simulink model "Ch12_PID_Simulink_Model"  (R2013b)
settings: Solver=ode45  StartTime=0.0  StopTime=100  MaxStep=0.1  RelTol=1e-3
libraries: simulink x1
settings Model: Creator=jeff  LastModifiedBy=jeff
settings DataIOCC: SignalLoggingSaveFormat=ModelDataLogs
settings OptimizationCC: ExpressionDepthLimit=2147483647
settings DebuggingCC: FcnCallInpInsideContextMsg=EnableAllAsWarning  StateNameClashWarn=warning

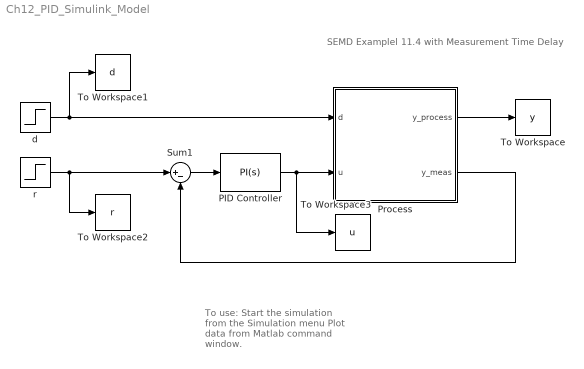
== system Ch12_PID_Simulink_Model ==
  note: SEMD Examplel 11.4 with Measurement Time Delay
  note: To use:
      |     Start the simulation from the Simulation menu
      |     Plot data from Matlab command window.
  PID Controller : simulink/Continuous/PID Controller  Controller=PI  TimeDomain=Continuous-time  SampleTime=1  IntegratorMethod=Forward Euler  FilterMethod=Forward Euler  Form=Ideal  P=1.12313558262161  I=0.142143488109628  D=0  N=100  InitialConditionSource=internal  InitialConditionForIntegrator=0  InitialConditionForFilter=0  ExternalReset=none  LimitOutput=off  UpperSaturationLimit=inf  LowerSaturationLimit=-inf  LinearizeAsGain=off  AntiWindupMode=none  Kb=1  TrackingMode=off  Kt=1  PParamMin=[]  PParamMax=[]  IParamMin=[]  IParamMax=[]  DParamMin=[]  DParamMax=[]  NParamMin=[]  NParamMax=[]  KbParamMin=[]  KbParamMax=[]  KtParamMin=[]  KtParamMax=[]  POutMin=[]  POutMax=[]  IOutMin=[]  IOutMax=[]  DOutMin=[]  DOutMax=[]  NOutMin=[]  NOutMax=[]  KbOutMin=[]  KbOutMax=[]  KtOutMin=[]  KtOutMax=[]  IntegratorOutMin=[]  IntegratorOutMax=[]  FilterOutMin=[]  FilterOutMax=[]  SumOutMin=[]  SumOutMax=[]  SumI1OutMin=[]  SumI1OutMax=[]  SumI2OutMin=[]  SumI2OutMax=[]  SumI3OutMin=[]  SumI3OutMax=[]  SumDOutMin=[]  SumDOutMax=[]  SaturationOutMin=[]  SaturationOutMax=[]  IntegratorContinuousStateAttributes=''  IntegratorStateMustResolveToSignalObject=off  IntegratorRTWStateStorageClass=Auto  FilterContinuousStateAttributes=''  FilterStateMustResolveToSignalObject=off  FilterRTWStateStorageClass=Auto
  Process : Subsystem
  Sum1 : Sum  Inputs=|+-
  To Workspace : ToWorkspace  VariableName=y  SampleTime=-1  SaveFormat=Timeseries
  To Workspace1 : ToWorkspace  VariableName=d  SampleTime=-1  SaveFormat=Timeseries
  To Workspace2 : ToWorkspace  VariableName=r  SampleTime=-1  SaveFormat=Timeseries
  To Workspace3 : ToWorkspace  VariableName=u  SampleTime=-1  SaveFormat=Timeseries
  d : Step  SampleTime=0
  r : Step  Time=50  SampleTime=0
  wires:
  d/1 -> To Workspace1/1, Process/1(d)
  r/1 -> To Workspace2/1, Sum1/1
  Process/2(y_meas) -> Sum1/2
  Sum1/1 -> PID Controller/1
  PID Controller/1 -> To Workspace3/1, Process/2(u)
  Process/1(y_process) -> To Workspace/1

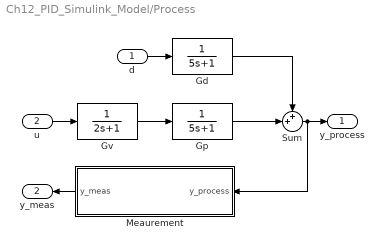
== system Ch12_PID_Simulink_Model/Process ==
  d : Inport
  u : Inport  Port=2
  Gd : TransferFcn  Denominator=[5 1]
  Gp : TransferFcn  Denominator=[5 1]
  Gv : TransferFcn  Denominator=[2 1]
  Meaurement : Subsystem
  Sum : Sum  Inputs=++|
  y_process : Outport
  y_meas : Outport  Port=2
  wires:
  Gv/1 -> Gp/1
  Sum/1 -> Meaurement/1(y_process), y_process/1
  Gd/1 -> Sum/1
  Gp/1 -> Sum/2
  d/1 -> Gd/1
  u/1 -> Gv/1
  Meaurement/1(y_meas) -> y_meas/1

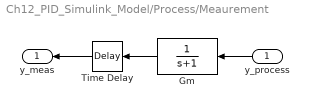
== system Ch12_PID_Simulink_Model/Process/Meaurement ==
  y_process : Inport
  Gm : TransferFcn  Denominator=[1 1]
  Time Delay : TransportDelay
  y_meas : Outport
  wires:
  Gm/1 -> Time Delay/1
  y_process/1 -> Gm/1
  Time Delay/1 -> y_meas/1
